simulink library "microgridLib"  (R2021b)
settings: Solver=VariableStepAuto  StartTime=0.0  StopTime=10.0  RelTol=1e-3
settings Model: Creator=Saad Khan  LastModifiedBy=Saad Khan

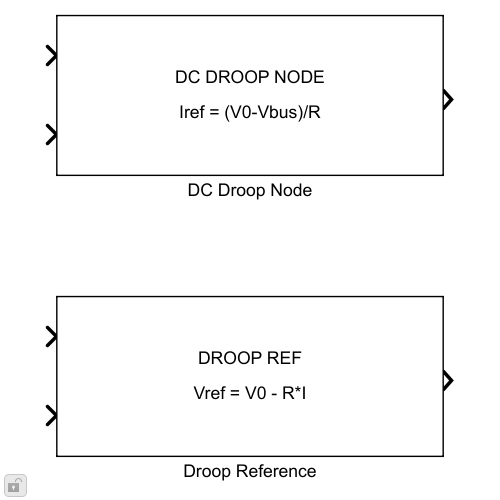
[thumbnail: Simulink's stored preview of the top-level diagram]
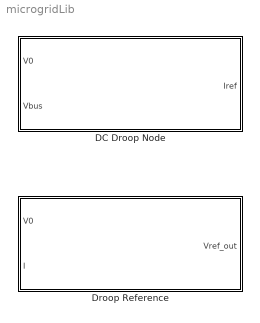
== system microgridLib ==
  DC Droop Node : Subsystem  mask{Rdroop=0.02, DB=0, Tf=3e-3, Imin=-inf, Imax=inf, Vinit=800}
      mask prompts: Rdroop "Droop slope R  [V per A]"; DB "Dead band half width  [V]"; Tf "Measurement filter time constant  [s]"; Imin "Minimum current  [A]"; Imax "Maximum current  [A]"; Vinit "Filter initial value  [V]"
      mask help:
      | Decentralised DC droop node.
      |
      |    Iref = sat( deadband( V0 - LPF(Vbus) ) / R )
      |
      | Pure proportional statism.  The node reads ONLY the DC bus voltage, so the
      | converters need no communication link between them - the bus voltage is the
      | communication.  At steady state the bus settles at  Vbus = V0 - R*Iref , and
      | it is that slope which shares load between parallel units.
      |
      | There is deliberately no integrator.  Two integrating units in parallel would
      | each force the bus to their own set-point and fight, and exact regulation
      | would destroy the sharing droop exists to provide.  The bus is expected to
      | sag under load, by design.
      |
      | R  slope, sized so the unit reaches rated current at the allowed deviation
      | DB dead band, keeps a unit out until higher-priority units are saturated
      | Tf measurement filter, separates droop from the fast inner current loop
      |
      | V0 is an INPUT, not a parameter, so a supervisor can shift the set-point
      | at run time (Phase 4: SOC target, island vs grid-connected).
      mask Display: disp('DC DROOP NODE\n\nIref = (V0-Vbus)/R')
  Droop Reference : Subsystem  mask{Rdroop=0.08, Vmin=0, Vmax=inf}
      mask prompts: Rdroop "Droop slope R  [V per A]"; Vmin "Minimum reference  [V]"; Vmax "Maximum reference  [V]"
      mask help:
      | Droop applied to a voltage set-point.
      |
      |    Vref = sat( V0 - R*I )
      |
      | For a converter that already regulates the bus with its own voltage loop
      | (the PV boost in voltage-control mode): drooping its set-point makes it
      | share instead of trying to hold one stiff voltage.  Used from Phase 4.
      mask Display: disp('DROOP REF\n\nVref = V0 - R*I')

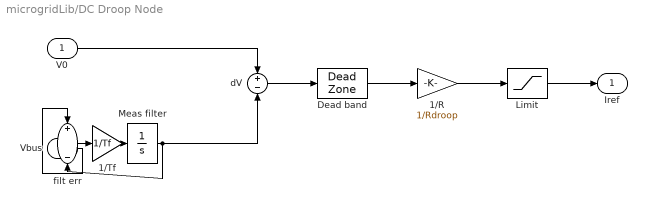
== system microgridLib/DC Droop Node ==
  V0 : Inport
  Vbus : Inport  Port=2
  1/R : Gain  Gain=1/Rdroop
  1/Tf : Gain  Gain=1/Tf
  Dead band : DeadZone  LowerValue=-DB  UpperValue=DB  SaturateOnIntegerOverflow=on
  Limit : Saturate  UpperLimit=Imax  LowerLimit=Imin
  Meas filter : Integrator  InitialCondition=Vinit
  dV : Sum  Inputs=+-
  filt err : Sum  Inputs=+-
  Iref : Outport
  wires:
  V0/1 -> dV/1
  dV/1 -> Dead band/1
  Dead band/1 -> 1/R/1
  1/R/1 -> Limit/1
  Limit/1 -> Iref/1
  Vbus/1 -> filt err/1
  filt err/1 -> 1/Tf/1
  1/Tf/1 -> Meas filter/1
  Meas filter/1 -> dV/2, filt err/2

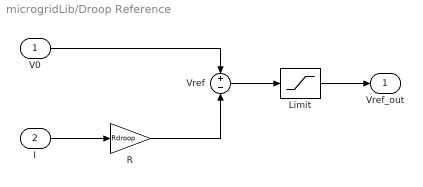
== system microgridLib/Droop Reference ==
  V0 : Inport
  I : Inport  Port=2
  Limit : Saturate  UpperLimit=Vmax  LowerLimit=Vmin
  R : Gain  Gain=Rdroop
  Vref : Sum  Inputs=+-
  Vref_out : Outport
  wires:
  V0/1 -> Vref/1
  I/1 -> R/1
  R/1 -> Vref/2
  Vref/1 -> Limit/1
  Limit/1 -> Vref_out/1
